simulink model "phase3PFDFinal"  (R2021a)
settings: Solver=VariableStepAuto  StartTime=0.0  StopTime=0.15  RelTol=1e-3
libraries: spsMosfetLib x4, spsVoltageMeasurementLib x2, spsDCVoltageSourceLib x1, spsCurrentMeasurementLib x1, spsSeriesRLCLoadLib x1, spspowerguiLib x1
settings Model: Creator=ishit  LastModifiedBy=user
settings SolverCC: AlgebraicLoopSolver=TrustRegion
settings DebuggingCC: SFMachineParentedDataDiag=warning

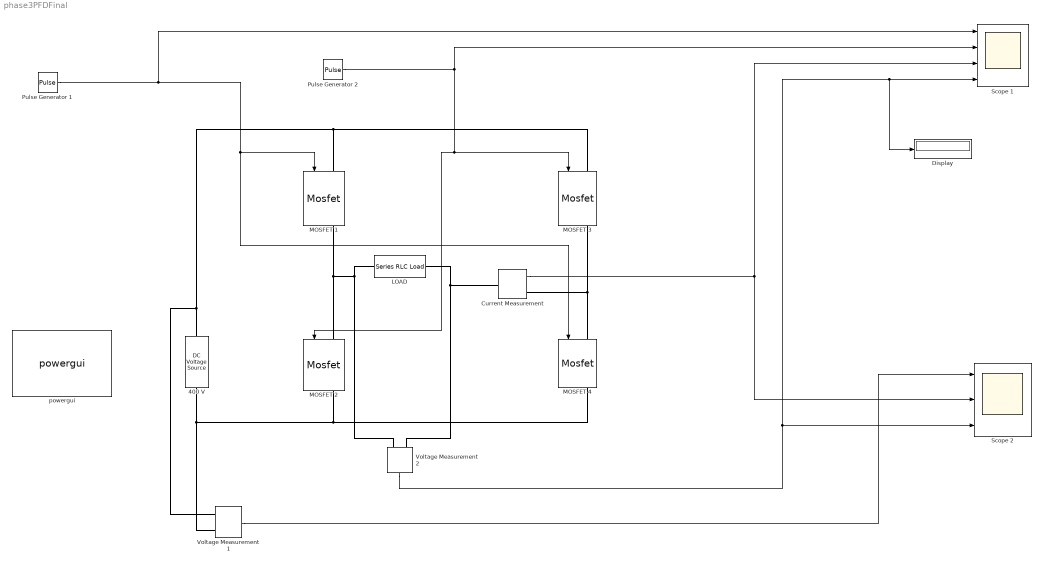
== system phase3PFDFinal ==
  400 V : spsDCVoltageSourceLib/DC Voltage Source  Amplitude=400  Measurements=None
  "Current Measurement " : spsCurrentMeasurementLib/Current Measurement  PhasorSimulation=off  OutputType=Complex  PSBequivalent=0
  Display : Display
  LOAD : spsSeriesRLCLoadLib/Series RLC Load  LConnTagsString=a  RConnTagsString=__new0  NominalVoltage=400  NominalFrequency=50  ActivePower=1500  InductivePower=0  CapacitivePower=0  Setx0=off  InitialVoltage=0  SetiL0=off  InitialCurrent=0  Measurements=None  LoadType=constant Z
  MOSFET {1..4} (4 alike) : spsMosfetLib/Mosfet  Ron=0.1  Lon=0  Rd=0.01  Vfd=0  IC=0  Rs=1e5  Cs=inf  Measurements=on
  Pulse Generator 1 : DiscretePulseGenerator  PulseType=Time based  Amplitude=5  Period=20e-3  PulseWidth=50
  Pulse Generator 2 : DiscretePulseGenerator  PulseType=Time based  Amplitude=5  Period=20e-3  PulseWidth=50  PhaseDelay=10e-3
  Scope 1 : Scope  NumInputPorts=4
  Scope 2 : Scope  NumInputPorts=3
  Voltage Measurement 1 : spsVoltageMeasurementLib/Voltage Measurement  PhasorSimulation=off  OutputType=Complex  PSBequivalent=0
  Voltage Measurement 2 : spsVoltageMeasurementLib/Voltage Measurement  PhasorSimulation=off  OutputType=Complex  PSBequivalent=0
  powergui : spspowerguiLib/powergui  Priority=1  SimulationMode=Continuous  SampleTime=50e-6  frequency=60  Iterations=50  frequencyindice=0  Pbase=100e6  ErrMax=1e-4  UnitsV=kV  UnitsW=MW  buscounter=0  FunctionMessages=off  echomessages=off  EnableUseOfTLC=off  CurrentSourceSwitches=off  DisableSnubberDevices=off  DisableRonSwitches=off  DisableVfSwitches=off  DisplayEquations=off  AutomaticDiscreteSolvers=off  SolverType=Tustin/Backward Euler (TBE)  Interpol=off  ExternalGateDelay=off  methode=off  Ts=100  x0status=blocks  SPID=on  SwTol=0  HookPort=off  NonlinearTolerance=1e-4  nMaxIteration=100  ContinueOnMaxIteration=off  RestoreLinks=warning  ResistiveCurrentMeasurement=off  Frange=[0:2:500]  Ylog=off  Xlog=on  ShowGrid=off  save=off  variable=ZData  structure=0  ZoomFFT=off  StartTime=0.0  cycles=1  DisplayStyle=1  fundamental=60  FreqAxis=off  MaxFrequency=1000  frequencyindicesteady=1  RmsSteady=1  display=off
  wires:
  Pulse Generator 2/1 -> MOSFET 2/1, MOSFET 3/1, Scope 1/2
  Pulse Generator 1/1 -> Scope 1/1, MOSFET 4/1, MOSFET 1/1
  Voltage Measurement 2/1 -> Display/1, Scope 1/4, Scope 2/3
  "Current Measurement "/1 -> Scope 1/3, Scope 2/2
  Voltage Measurement 1/1 -> Scope 2/1
  connections:
  MOSFET 1/RConn1 -- Voltage Measurement 2/LConn1 -- LOAD/LConn1 -- MOSFET 2/LConn1
  MOSFET 3/RConn1 -- "Current Measurement "/RConn1 -- MOSFET 4/LConn1
  MOSFET 2/RConn1 -- 400 V/LConn1 -- Voltage Measurement 1/LConn2 -- MOSFET 4/RConn1
  MOSFET 1/LConn1 -- Voltage Measurement 1/LConn1 -- 400 V/RConn1 -- MOSFET 3/LConn1
  "Current Measurement "/LConn1 -- LOAD/RConn1 -- Voltage Measurement 2/LConn2
